simulink model "PTCOP_TrqCnv"  (R2016b)
settings: configuration reference "CodeGenConfigSet" (kept outside this file)
libraries: CXLib x6
settings Model: Creator=Wollf  LastModifiedBy=yangyang
settings ConfigSetRef: SourceLocation=Base Workspace

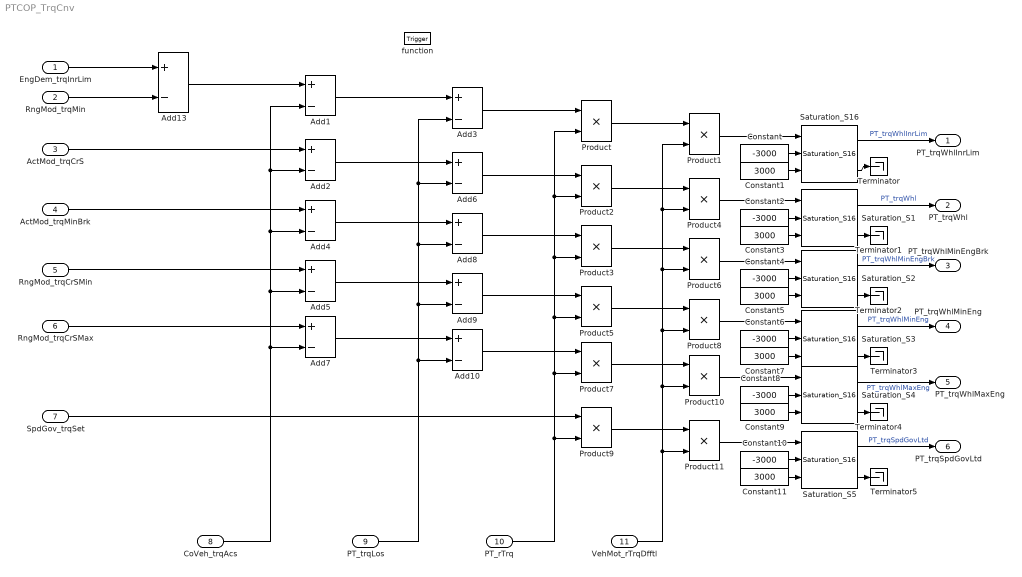
== system PTCOP_TrqCnv ==
  EngDem_trqInrLim : Inport  Tag=Nm  Description=Resulting limiting torque (inner engine torque)  OutMin=-3276.8  OutMax=3276.7  OutDataTypeStr=Trq_Nm
  RngMod_trqMin : Inport  Tag=Nm  Description=Drag torque (minimum torque)  Port=2  OutMin=-3276.8  OutMax=3276.7  OutDataTypeStr=Trq_Nm
  ActMod_trqCrS : Inport  Tag=Nm  Description=Current crankshaft torque  Port=3  OutMin=-3276.8  OutMax=3276.7  OutDataTypeStr=Trq_Nm
  ActMod_trqMinBrk : Inport  Tag=Nm  Description=minimum possible drag torque  Port=4  OutMin=-3276.8  OutMax=3276.7  OutDataTypeStr=Trq_Nm
  RngMod_trqCrSMin : Inport  Tag=Nm  Description=minimal crankshaft torque  Port=5  OutMin=-3276.8  OutMax=3276.7  OutDataTypeStr=Trq_Nm
  RngMod_trqCrSMax : Inport  Tag=Nm  Description=maximal crankshaft torque  Port=6  OutMin=-3276.8  OutMax=3276.7  OutDataTypeStr=Trq_Nm
  SpdGov_trqSet : Inport  Tag=Nm  Description=Set point torque of SpdGov on the fuel path  Port=7  OutMin=-3000  OutMax=3000  OutDataTypeStr=Trq_Nm
  CoVeh_trqAcs : Inport  Tag=Nm  Description=message for demand of accessories  Port=8  OutMin=-3276.8  OutMax=3276.7  OutDataTypeStr=Trq_Nm
  PT_trqLos : Inport  Tag=Nm  Description=Parameter for loss torque of the drive train  Port=9  OutMin=-3000  OutMax=3000  OutDataTypeStr=Trq_Nm
  PT_rTrq : Inport  Description=Powertrain torque ratio  Port=10  OutMin=-100  OutMax=100  OutDataTypeStr=TransRatio
  VehMot_rTrqDfftl : Inport  Description=Torque ratio of differential  Port=11  OutMin=-300  OutMax=300  OutDataTypeStr=TransRatio
  function : TriggerPort  TriggerType=function-call  VariantControl=Variant
  Add{1..10,13} (11 alike) : Sum  Inputs=+-  SaturateOnIntegerOverflow=on  InputSameDT=on
  Constant{,2,4,6,8,10} (6 alike) : Constant  Value=-3000  OutDataTypeStr=Inherit: Inherit via back propagation
  Constant{1,3,5,7,9,11} (6 alike) : Constant  Value=3000  OutDataTypeStr=Inherit: Inherit via back propagation
  Product{,1..11} (12 alike) : Product  OutDataTypeStr=Trq_Nm  RndMeth=Round  SaturateOnIntegerOverflow=on
  Saturation_S{1..5,16} (6 alike) : CXLib/Saturation_S16
  Terminator{,1..5} (6 alike) : Terminator
  PT_trqWhlInrLim : Outport  Tag=Nm  Description=Engine torque limitation converted to wheel torque  OutMin=-3000  OutMax=3000  OutDataTypeStr=Trq_Nm
  PT_trqWhl : Outport  Tag=Nm  Description=Actual wheel torque  Port=2  OutMin=-3000  OutMax=3000  OutDataTypeStr=Trq_Nm
  PT_trqWhlMinEngBrk : Outport  Tag=Nm  Description=Minimum possible drag torque  Port=3  OutMin=-3000  OutMax=3000  OutDataTypeStr=Trq_Nm
  PT_trqWhlMinEng : Outport  Tag=Nm  Description=Minimum wheel torque from the engine  Port=4  OutMin=-3000  OutMax=3000  OutDataTypeStr=Trq_Nm
  PT_trqWhlMaxEng : Outport  Tag=Nm  Description=Maximum wheel torque from the engine  Port=5  OutMin=-3000  OutMax=3000  OutDataTypeStr=Trq_Nm
  PT_trqSpdGovLtd : Outport  Tag=Nm  Description=Low-idle governor torque  Port=6  OutMin=-3000  OutMax=3000  OutDataTypeStr=Trq_Nm
  wires:
  VehMot_rTrqDfftl/1 -> Product11/2, Product10/2, Product8/2, Product6/2, Product4/2, Product1/2
  PT_rTrq/1 -> Product9/2, Product7/2, Product5/2, Product3/2, Product2/2, Product/2
  Add1/1 -> Add3/1
  Add13/1 -> Add1/1
  ActMod_trqMinBrk/1 -> Add4/1
  Add4/1 -> Add8/1
  Product3/1 -> Product6/1
  Add8/1 -> Product3/1
  EngDem_trqInrLim/1 -> Add13/1
  Product9/1 -> Product11/1
  SpdGov_trqSet/1 -> Product9/1
  CoVeh_trqAcs/1 -> Add7/2, Add5/2, Add4/2, Add2/2, Add1/2
  Product5/1 -> Product8/1
  Add5/1 -> Add9/1
  RngMod_trqCrSMin/1 -> Add5/1
  Add9/1 -> Product5/1
  RngMod_trqCrSMax/1 -> Add7/1
  Add7/1 -> Add10/1
  Add10/1 -> Product7/1
  Product7/1 -> Product10/1
  RngMod_trqMin/1 -> Add13/2
  Product/1 -> Product1/1
  Add2/1 -> Add6/1
  Add6/1 -> Product2/1
  ActMod_trqCrS/1 -> Add2/1
  Product2/1 -> Product4/1
  Add3/1 -> Product/1
  PT_trqLos/1 -> Add10/2, Add9/2, Add8/2, Add6/2, Add3/2
  Saturation_S16/1 -> PT_trqWhlInrLim/1  "PT_trqWhlInrLim"
  Saturation_S1/1 -> PT_trqWhl/1  "PT_trqWhl"
  Saturation_S2/1 -> PT_trqWhlMinEngBrk/1  "PT_trqWhlMinEngBrk"
  Saturation_S3/1 -> PT_trqWhlMinEng/1  "PT_trqWhlMinEng"
  Saturation_S4/1 -> PT_trqWhlMaxEng/1  "PT_trqWhlMaxEng"
  Saturation_S5/1 -> PT_trqSpdGovLtd/1  "PT_trqSpdGovLtd"
  Saturation_S16/2 -> Terminator/1
  Constant/1 -> Saturation_S16/2
  Constant1/1 -> Saturation_S16/3
  Product1/1 -> Saturation_S16/1
  Saturation_S1/2 -> Terminator1/1
  Constant2/1 -> Saturation_S1/2
  Constant3/1 -> Saturation_S1/3
  Product4/1 -> Saturation_S1/1
  Saturation_S2/2 -> Terminator2/1
  Constant4/1 -> Saturation_S2/2
  Constant5/1 -> Saturation_S2/3
  Product6/1 -> Saturation_S2/1
  Saturation_S3/2 -> Terminator3/1
  Constant6/1 -> Saturation_S3/2
  Constant7/1 -> Saturation_S3/3
  Product8/1 -> Saturation_S3/1
  Saturation_S4/2 -> Terminator4/1
  Constant8/1 -> Saturation_S4/2
  Constant9/1 -> Saturation_S4/3
  Product10/1 -> Saturation_S4/1
  Saturation_S5/2 -> Terminator5/1
  Constant10/1 -> Saturation_S5/2
  Constant11/1 -> Saturation_S5/3
  Product11/1 -> Saturation_S5/1
